simulink model "holdImageProcessing"  (R2018b)
settings: Solver=FixedStepAuto  StartTime=0.0  StopTime=70  FixedStep=0.025  RelTol=1e-3  EnableMultiTasking=on
settings Model: Creator=Andy  LastModifiedBy=Andy
settings SolverCC: PositivePriorityOrder=on
settings DataIOCC: Decimation=5  SaveFormat=StructureWithTime
settings OptimizationCC: EnhancedBackFolding=on  PassReuseOutputArgsAs=Individual arguments  MaxStackSize=64  OptimizeBlockOrder=speed  DifferentSizesBufferReuse=on  OptimizationCustomize=off
settings DebuggingCC: ParameterTunabilityLossMsg=error
settings HardwareCC: ProdBitPerPointer=32  ProdBitPerSizeT=32  ProdBitPerPtrDiffT=32  ProdLargestAtomicInteger=Long  ProdLargestAtomicFloat=Double  ProdWordSize=32  ProdHWDeviceType=ARM Compatible->ARM Cortex
settings ModelReferenceCC: ModelReferenceNumInstancesAllowed=Single
settings RTWCC: SystemTargetFile=ert.tlc  HardwareBoard=Raspberry Pi  TLCOptions="-aInlineSetEventsForThisBaseRateFcn=TLC_FALSE -aSuppressMultiTaskScheduler=TLC_FALSE  -aRateBasedStepFcn=0"  GenCodeOnly=on  TemplateMakefile=ert_default_tmf  GenerateReport=on  Toolchain=GNU GCC Raspberry Pi  BuildConfiguration=Faster Runs  IncludeHyperlinkInReport=on  LaunchReport=on  TargetLang=C++  GenerateTraceInfo=on  GenerateTraceReport=on  GenerateTraceReportSl=on  GenerateTraceReportSf=on  GenerateTraceReportEml=on
settings CodeAppCC: ForceParamTrailComments=on  IgnoreCustomStorageClasses=off  OperatorAnnotations=on  SimulinkDataObjDesc=on  SFDataObjDesc=on  InsertBlockDesc=on
settings ERTTargetCC: TargetLangStandard=C++03 (ISO)  MatFileLogging=on  MultiInstanceERTCode=on  CodeInterfacePackaging=C++ class  SupportVariableSizeSignals=on  MultiInstanceErrorCode=Warning  RootIOFormat=Structure reference

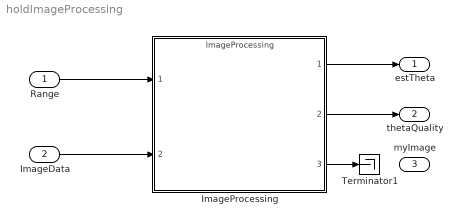
== system holdImageProcessing ==
  Range : Inport  OutDataTypeStr=double  PortDimensions=4
  ImageData : Inport  Port=2  OutDataTypeStr=uint8  PortDimensions=[307200]
  ImageProcessing : ModelReference  ModelNameDialog=ImageProcessing  SimulationMode=Normal  ModelReferenceVersion=1.5
  Terminator1 : Terminator
  estTheta : Outport  OutDataTypeStr=double  PortDimensions=1
  thetaQuality : Outport  Port=2  OutDataTypeStr=double  PortDimensions=1
  myImage : Outport  Port=3  OutDataTypeStr=uint8
  wires:
  Range/1 -> ImageProcessing/1
  ImageData/1 -> ImageProcessing/2
  ImageProcessing/1 -> estTheta/1
  ImageProcessing/2 -> thetaQuality/1
  ImageProcessing/3 -> Terminator1/1
